simulink model "GPCA_Alarm"  (Simulink 8.7)
settings: Solver=VariableStepAuto  StartTime=0.0  StopTime=10.0  RelTol=1e-3
libraries: simulink x14
(part 1 of 3)
settings Model: Creator=bourbouh  LastModifiedBy=bourbouh
settings DataIOCC: LimitDataPoints=off  SaveFormat=Dataset
settings DebuggingCC: UnderspecifiedInitializationDetection=Simplified  MergeDetectMultiDrivingBlocksExec=error
settings HardwareCC: ProdBitPerPointer=64  ProdLargestAtomicFloat=Float  ProdIntDivRoundTo=Zero  ProdEndianess=LittleEndian  ProdWordSize=64  ProdHWDeviceType=Intel->x86-64 (Windows64)
settings ModelReferenceCC: PropagateSignalLabelsOutOfModel=on
settings ConfigComp: CovModelRefEnable=off

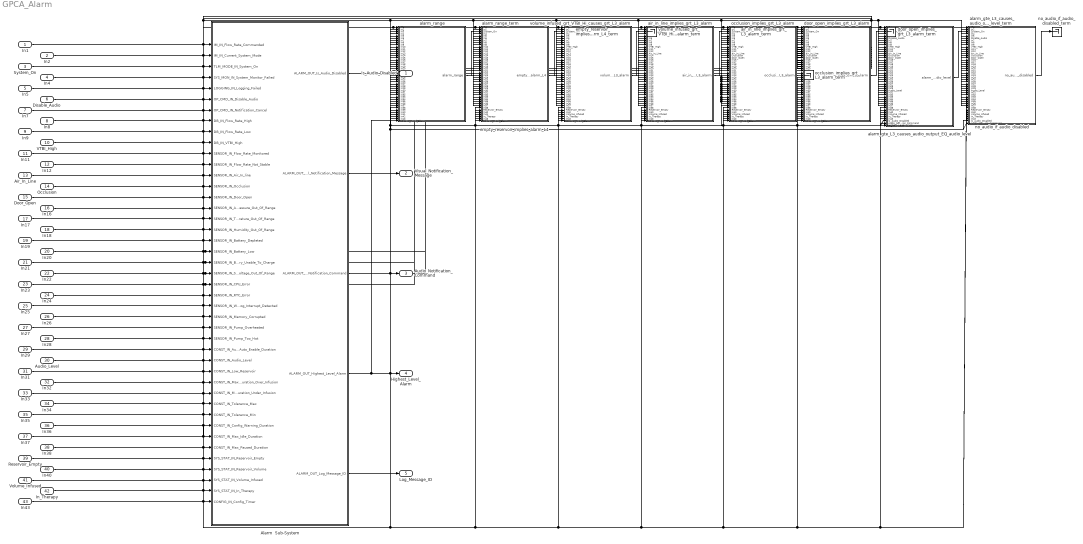
== system GPCA_Alarm ==
  In1 : Inport
  In2 : Inport  Port=2
  System_On : Inport  Port=3
  In4 : Inport  Port=4
  In5 : Inport  Port=5
  Disable_Audio : Inport  Port=6
  In7 : Inport  Port=7
  In8 : Inport  Port=8
  In9 : Inport  Port=9
  VTBI_High : Inport  Port=10
  In11 : Inport  Port=11
  In12 : Inport  Port=12
  Air_In_Line : Inport  Port=13
  Occlusion : Inport  Port=14
  Door_Open : Inport  Port=15
  In16 : Inport  Port=16
  In17 : Inport  Port=17
  In18 : Inport  Port=18
  In19 : Inport  Port=19
  In20 : Inport  Port=20
  In21 : Inport  Port=21
  In22 : Inport  Port=22
  In23 : Inport  Port=23
  In24 : Inport  Port=24
  In25 : Inport  Port=25
  In26 : Inport  Port=26
  In27 : Inport  Port=27
  In28 : Inport  Port=28
  In29 : Inport  Port=29
  Audio_Level : Inport  Port=30
  In31 : Inport  Port=31
  In32 : Inport  Port=32
  In33 : Inport  Port=33
  In34 : Inport  Port=34
  In35 : Inport  Port=35
  In36 : Inport  Port=36
  In37 : Inport  Port=37
  In38 : Inport  Port=38
  Reservoir_Empty : Inport  Port=39
  In40 : Inport  Port=40
  Volume_Infused : Inport  Port=41
  In_Therapy : Inport  Port=42
  In43 : Inport  Port=43
  Alarm  Sub-System : Stateflow chart  TreatAsAtomicUnit=on
  air_in_line_implies_grt_L3_alarm : Subsystem  TreatAsAtomicUnit=on  mask(Observer){AnnotationType=ensures, ObserverType=[]}
      mask prompts: AnnotationType "Type of annotation (pre/post...)"; ObserverType "Observer type"
      mask help:
      | Set an observer for the system.
      | The annotation type parameter sets the type of observer:
      | - requires : pre-condition
      | - ensures : post-condition
      | - assert : an assertion
      | - observer : the observer computes a special type of properties
      mask TypeOptions AnnotationType: ensures | requires | assert | observer
      mask Callback AnnotationType:
      | paramStr = get_param(gcb, 'MaskValues');
      | if strcmp(paramStr{1}(1),'o')
      | set_param(gcb,'MaskVisibilities',{'on';'on'});
      | paramStr{2} = 'ellipsoid';
      | set_param(gcb,'MaskValues',paramStr);
      | else
      | set_param(gcb,'MaskVisibilities',{'on';'off'});
      | end
      | clear paramStr;
      mask Callback ObserverType:
      | paramStr = get_param(gcb, 'MaskValues');
      | if strcmp(paramStr{1}(1),'o')
      | set_param(gcb,'MaskVisibilities',{'on';'on'});
      | paramStr{2} = 'ellipsoid';
      | set_param(gcb,'MaskValues',paramStr);
      | else
      | set_param(gcb,'MaskVisibilities',{'on';'off'});
      | end
      | clear paramStr;
      mask Display:
      | color('black')
      | text(0.5, 0.5, ['Property: ''' get_param(gcb,'name') ''''], 'horizontalAlignment', 'center');
      | text(0.99, 0.03, '{\bf\fontsize{12}TIMEOUT}', 'hor', 'right', 'ver', 'bottom', 'texmode', 'on');
  air_in_line_implies_grt_L3_alarm_term : Terminator
  alarm_gte_L3_causes_audio_output_EQ_audio_level : Subsystem  TreatAsAtomicUnit=on  mask(Observer){AnnotationType=ensures, ObserverType=[]}
      mask prompts: AnnotationType "Type of annotation (pre/post...)"; ObserverType "Observer type"
      mask help:
      | Set an observer for the system.
      | The annotation type parameter sets the type of observer:
      | - requires : pre-condition
      | - ensures : post-condition
      | - assert : an assertion
      | - observer : the observer computes a special type of properties
      mask TypeOptions AnnotationType: ensures | requires | assert | observer
      mask Callback AnnotationType:
      | paramStr = get_param(gcb, 'MaskValues');
      | if strcmp(paramStr{1}(1),'o')
      | set_param(gcb,'MaskVisibilities',{'on';'on'});
      | paramStr{2} = 'ellipsoid';
      | set_param(gcb,'MaskValues',paramStr);
      | else
      | set_param(gcb,'MaskVisibilities',{'on';'off'});
      | end
      | clear paramStr;
      mask Callback ObserverType:
      | paramStr = get_param(gcb, 'MaskValues');
      | if strcmp(paramStr{1}(1),'o')
      | set_param(gcb,'MaskVisibilities',{'on';'on'});
      | paramStr{2} = 'ellipsoid';
      | set_param(gcb,'MaskValues',paramStr);
      | else
      | set_param(gcb,'MaskVisibilities',{'on';'off'});
      | end
      | clear paramStr;
      mask Display:
      | color('red')
      | text(0.5, 0.5, ['CoCoSpec: ''' get_param(gcb,'name') ''''], 'horizontalAlignment', 'center');
      | text(0.99, 0.03, '{\bf\fontsize{12}TO BE VERIFIED}', 'hor', 'right', 'ver', 'bottom', 'texmode', 'on');
  alarm_gte_L3_causes_audio_output_EQ_audio_level_term : Terminator
  alarm_range : Subsystem  TreatAsAtomicUnit=on  mask(Observer){AnnotationType=ensures, ObserverType=[]}
      mask prompts: AnnotationType "Type of annotation (pre/post...)"; ObserverType "Observer type"
      mask help:
      | Set an observer for the system.
      | The annotation type parameter sets the type of observer:
      | - requires : pre-condition
      | - ensures : post-condition
      | - assert : an assertion
      | - observer : the observer computes a special type of properties
      mask TypeOptions AnnotationType: ensures | requires | assert | observer
      mask Callback AnnotationType:
      | paramStr = get_param(gcb, 'MaskValues');
      | if strcmp(paramStr{1}(1),'o')
      | set_param(gcb,'MaskVisibilities',{'on';'on'});
      | paramStr{2} = 'ellipsoid';
      | set_param(gcb,'MaskValues',paramStr);
      | else
      | set_param(gcb,'MaskVisibilities',{'on';'off'});
      | end
      | clear paramStr;
      mask Callback ObserverType:
      | paramStr = get_param(gcb, 'MaskValues');
      | if strcmp(paramStr{1}(1),'o')
      | set_param(gcb,'MaskVisibilities',{'on';'on'});
      | paramStr{2} = 'ellipsoid';
      | set_param(gcb,'MaskValues',paramStr);
      | else
      | set_param(gcb,'MaskVisibilities',{'on';'off'});
      | end
      | clear paramStr;
      mask Display:
      | color('black')
      | text(0.5, 0.5, ['Property: ''' get_param(gcb,'name') ''''], 'horizontalAlignment', 'center');
      | text(0.99, 0.03, '{\bf\fontsize{12}SAFE}', 'hor', 'right', 'ver', 'bottom', 'texmode', 'on');
  alarm_range_term : Terminator
  door_open_implies_grt_L3_alarm : Subsystem  TreatAsAtomicUnit=on  mask(Observer){AnnotationType=ensures, ObserverType=[]}
      mask prompts: AnnotationType "Type of annotation (pre/post...)"; ObserverType "Observer type"
      mask help:
      | Set an observer for the system.
      | The annotation type parameter sets the type of observer:
      | - requires : pre-condition
      | - ensures : post-condition
      | - assert : an assertion
      | - observer : the observer computes a special type of properties
      mask TypeOptions AnnotationType: ensures | requires | assert | observer
      mask Callback AnnotationType:
      | paramStr = get_param(gcb, 'MaskValues');
      | if strcmp(paramStr{1}(1),'o')
      | set_param(gcb,'MaskVisibilities',{'on';'on'});
      | paramStr{2} = 'ellipsoid';
      | set_param(gcb,'MaskValues',paramStr);
      | else
      | set_param(gcb,'MaskVisibilities',{'on';'off'});
      | end
      | clear paramStr;
      mask Callback ObserverType:
      | paramStr = get_param(gcb, 'MaskValues');
      | if strcmp(paramStr{1}(1),'o')
      | set_param(gcb,'MaskVisibilities',{'on';'on'});
      | paramStr{2} = 'ellipsoid';
      | set_param(gcb,'MaskValues',paramStr);
      | else
      | set_param(gcb,'MaskVisibilities',{'on';'off'});
      | end
      | clear paramStr;
      mask Display:
      | color('black')
      | text(0.5, 0.5, ['Property: ''' get_param(gcb,'name') ''''], 'horizontalAlignment', 'center');
      | text(0.99, 0.03, '{\bf\fontsize{12}TIMEOUT}', 'hor', 'right', 'ver', 'bottom', 'texmode', 'on');
  door_open_implies_grt_L3_alarm_term : Terminator
  empty_reservoir_implies_alarm_L4 : Subsystem  TreatAsAtomicUnit=on  mask(Observer){AnnotationType=ensures, ObserverType=[]}
      mask prompts: AnnotationType "Type of annotation (pre/post...)"; ObserverType "Observer type"
      mask help:
      | Set an observer for the system.
      | The annotation type parameter sets the type of observer:
      | - requires : pre-condition
      | - ensures : post-condition
      | - assert : an assertion
      | - observer : the observer computes a special type of properties
      mask TypeOptions AnnotationType: ensures | requires | assert | observer
      mask Callback AnnotationType:
      | paramStr = get_param(gcb, 'MaskValues');
      | if strcmp(paramStr{1}(1),'o')
      | set_param(gcb,'MaskVisibilities',{'on';'on'});
      | paramStr{2} = 'ellipsoid';
      | set_param(gcb,'MaskValues',paramStr);
      | else
      | set_param(gcb,'MaskVisibilities',{'on';'off'});
      | end
      | clear paramStr;
      mask Callback ObserverType:
      | paramStr = get_param(gcb, 'MaskValues');
      | if strcmp(paramStr{1}(1),'o')
      | set_param(gcb,'MaskVisibilities',{'on';'on'});
      | paramStr{2} = 'ellipsoid';
      | set_param(gcb,'MaskValues',paramStr);
      | else
      | set_param(gcb,'MaskVisibilities',{'on';'off'});
      | end
      | clear paramStr;
      mask Display:
      | color('black')
      | text(0.5, 0.5, ['Property: ''' get_param(gcb,'name') ''''], 'horizontalAlignment', 'center');
      | text(0.99, 0.03, '{\bf\fontsize{12}SAFE}', 'hor', 'right', 'ver', 'bottom', 'texmode', 'on');
  empty_reservoir_implies_alarm_L4_term : Terminator
  no_audio_if_audio_disabled : Subsystem  TreatAsAtomicUnit=on  mask(Observer){AnnotationType=ensures, ObserverType=[]}
      mask prompts: AnnotationType "Type of annotation (pre/post...)"; ObserverType "Observer type"
      mask help:
      | Set an observer for the system.
      | The annotation type parameter sets the type of observer:
      | - requires : pre-condition
      | - ensures : post-condition
      | - assert : an assertion
      | - observer : the observer computes a special type of properties
      mask TypeOptions AnnotationType: ensures | requires | assert | observer
      mask Callback AnnotationType:
      | paramStr = get_param(gcb, 'MaskValues');
      | if strcmp(paramStr{1}(1),'o')
      | set_param(gcb,'MaskVisibilities',{'on';'on'});
      | paramStr{2} = 'ellipsoid';
      | set_param(gcb,'MaskValues',paramStr);
      | else
      | set_param(gcb,'MaskVisibilities',{'on';'off'});
      | end
      | clear paramStr;
      mask Callback ObserverType:
      | paramStr = get_param(gcb, 'MaskValues');
      | if strcmp(paramStr{1}(1),'o')
      | set_param(gcb,'MaskVisibilities',{'on';'on'});
      | paramStr{2} = 'ellipsoid';
      | set_param(gcb,'MaskValues',paramStr);
      | else
      | set_param(gcb,'MaskVisibilities',{'on';'off'});
      | end
      | clear paramStr;
      mask Display:
      | color('red')
      | text(0.5, 0.5, ['CoCoSpec: ''' get_param(gcb,'name') ''''], 'horizontalAlignment', 'center');
      | text(0.99, 0.03, '{\bf\fontsize{12}TO BE VERIFIED}', 'hor', 'right', 'ver', 'bottom', 'texmode', 'on');
  no_audio_if_audio_disabled_term : Terminator
  occlusion_implies_grt_L3_alarm : Subsystem  TreatAsAtomicUnit=on  mask(Observer){AnnotationType=ensures, ObserverType=[]}
      mask prompts: AnnotationType "Type of annotation (pre/post...)"; ObserverType "Observer type"
      mask help:
      | Set an observer for the system.
      | The annotation type parameter sets the type of observer:
      | - requires : pre-condition
      | - ensures : post-condition
      | - assert : an assertion
      | - observer : the observer computes a special type of properties
      mask TypeOptions AnnotationType: ensures | requires | assert | observer
      mask Callback AnnotationType:
      | paramStr = get_param(gcb, 'MaskValues');
      | if strcmp(paramStr{1}(1),'o')
      | set_param(gcb,'MaskVisibilities',{'on';'on'});
      | paramStr{2} = 'ellipsoid';
      | set_param(gcb,'MaskValues',paramStr);
      | else
      | set_param(gcb,'MaskVisibilities',{'on';'off'});
      | end
      | clear paramStr;
      mask Callback ObserverType:
      | paramStr = get_param(gcb, 'MaskValues');
      | if strcmp(paramStr{1}(1),'o')
      | set_param(gcb,'MaskVisibilities',{'on';'on'});
      | paramStr{2} = 'ellipsoid';
      | set_param(gcb,'MaskValues',paramStr);
      | else
      | set_param(gcb,'MaskVisibilities',{'on';'off'});
      | end
      | clear paramStr;
      mask Display:
      | color('black')
      | text(0.5, 0.5, ['Property: ''' get_param(gcb,'name') ''''], 'horizontalAlignment', 'center');
      | text(0.99, 0.03, '{\bf\fontsize{12}TIMEOUT}', 'hor', 'right', 'ver', 'bottom', 'texmode', 'on');
  occlusion_implies_grt_L3_alarm_term : Terminator
  volume_infused_grt_VTBI_Hi_causes_grt_L3_alarm : Subsystem  TreatAsAtomicUnit=on  mask(Observer){AnnotationType=ensures, ObserverType=[]}
      mask prompts: AnnotationType "Type of annotation (pre/post...)"; ObserverType "Observer type"
      mask help:
      | Set an observer for the system.
      | The annotation type parameter sets the type of observer:
      | - requires : pre-condition
      | - ensures : post-condition
      | - assert : an assertion
      | - observer : the observer computes a special type of properties
      mask TypeOptions AnnotationType: ensures | requires | assert | observer
      mask Callback AnnotationType:
      | paramStr = get_param(gcb, 'MaskValues');
      | if strcmp(paramStr{1}(1),'o')
      | set_param(gcb,'MaskVisibilities',{'on';'on'});
      | paramStr{2} = 'ellipsoid';
      | set_param(gcb,'MaskValues',paramStr);
      | else
      | set_param(gcb,'MaskVisibilities',{'on';'off'});
      | end
      | clear paramStr;
      mask Callback ObserverType:
      | paramStr = get_param(gcb, 'MaskValues');
      | if strcmp(paramStr{1}(1),'o')
      | set_param(gcb,'MaskVisibilities',{'on';'on'});
      | paramStr{2} = 'ellipsoid';
      | set_param(gcb,'MaskValues',paramStr);
      | else
      | set_param(gcb,'MaskVisibilities',{'on';'off'});
      | end
      | clear paramStr;
      mask Display:
      | color('black')
      | text(0.5, 0.5, ['Property: ''' get_param(gcb,'name') ''''], 'horizontalAlignment', 'center');
      | text(0.99, 0.03, '{\bf\fontsize{12}SAFE}', 'hor', 'right', 'ver', 'bottom', 'texmode', 'on');
  volume_infused_grt_VTBI_Hi_causes_grt_L3_alarm_term : Terminator
  Is_Audio_Disabled : Outport
  Visual_Notification_Message : Outport  Port=2
  Audio_Notification_Command : Outport  Port=3
  Highest_Level_Alarm : Outport  Port=4
  Log_Message_ID : Outport  Port=5
  wires:
  In1/1 -> alarm_gte_L3_causes_audio_output_EQ_audio_level/1(In1), no_audio_if_audio_disabled/1(In1), door_open_implies_grt_L3_alarm/1(In1), occlusion_implies_grt_L3_alarm/1(In1), air_in_line_implies_grt_L3_alarm/1(In1), volume_infused_grt_VTBI_Hi_causes_grt_L3_alarm/1(In1), empty_reservoir_implies_alarm_L4/1(In1), alarm_range/1(In1), Alarm  Sub-System/1(IM_IN_Flow_Rate_Commanded)
  In2/1 -> alarm_gte_L3_causes_audio_output_EQ_audio_level/2(In2), no_audio_if_audio_disabled/2(In2), occlusion_implies_grt_L3_alarm/2(In2), air_in_line_implies_grt_L3_alarm/2(In2), volume_infused_grt_VTBI_Hi_causes_grt_L3_alarm/2(In2), empty_reservoir_implies_alarm_L4/2(In2), alarm_range/2(In2), door_open_implies_grt_L3_alarm/2(In2), Alarm  Sub-System/2(IM_IN_Current_System_Mode)
  System_On/1 -> alarm_gte_L3_causes_audio_output_EQ_audio_level/3(System_On), no_audio_if_audio_disabled/3(System_On), occlusion_implies_grt_L3_alarm/3(System_On), air_in_line_implies_grt_L3_alarm/3(System_On), volume_infused_grt_VTBI_Hi_causes_grt_L3_alarm/3(System_On), empty_reservoir_implies_alarm_L4/3(System_On), alarm_range/3(In3), door_open_implies_grt_L3_alarm/3(System_On), Alarm  Sub-System/3(TLM_MODE_IN_System_On)
  In4/1 -> alarm_gte_L3_causes_audio_output_EQ_audio_level/4(In4), no_audio_if_audio_disabled/4(In4), occlusion_implies_grt_L3_alarm/4(In4), air_in_line_implies_grt_L3_alarm/4(In4), volume_infused_grt_VTBI_Hi_causes_grt_L3_alarm/4(In4), empty_reservoir_implies_alarm_L4/4(In4), alarm_range/4(In4), door_open_implies_grt_L3_alarm/4(In4), Alarm  Sub-System/4(SYS_MON_IN_System_Monitor_Failed)
  In5/1 -> alarm_gte_L3_causes_audio_output_EQ_audio_level/5(In5), no_audio_if_audio_disabled/5(In5), occlusion_implies_grt_L3_alarm/5(In5), air_in_line_implies_grt_L3_alarm/5(In5), volume_infused_grt_VTBI_Hi_causes_grt_L3_alarm/5(In5), empty_reservoir_implies_alarm_L4/5(In5), alarm_range/5(In5), door_open_implies_grt_L3_alarm/5(In5), Alarm  Sub-System/5(LOGGING_IN_Logging_Failed)
  Disable_Audio/1 -> alarm_gte_L3_causes_audio_output_EQ_audio_level/6(Disable_Audio), no_audio_if_audio_disabled/6(Disable_Audio), occlusion_implies_grt_L3_alarm/6(In6), air_in_line_implies_grt_L3_alarm/6(In6), volume_infused_grt_VTBI_Hi_causes_grt_L3_alarm/6(In6), empty_reservoir_implies_alarm_L4/6(In6), alarm_range/6(In6), door_open_implies_grt_L3_alarm/6(In6), Alarm  Sub-System/6(OP_CMD_IN_Disable_Audio)
  In7/1 -> alarm_gte_L3_causes_audio_output_EQ_audio_level/7(In7), no_audio_if_audio_disabled/7(In7), occlusion_implies_grt_L3_alarm/7(In7), air_in_line_implies_grt_L3_alarm/7(In7), volume_infused_grt_VTBI_Hi_causes_grt_L3_alarm/7(In7), empty_reservoir_implies_alarm_L4/7(In7), alarm_range/7(In7), door_open_implies_grt_L3_alarm/7(In7), Alarm  Sub-System/7(OP_CMD_IN_Notification_Cancel)
  In8/1 -> alarm_gte_L3_causes_audio_output_EQ_audio_level/8(In8), no_audio_if_audio_disabled/8(In8), occlusion_implies_grt_L3_alarm/8(In8), air_in_line_implies_grt_L3_alarm/8(In8), volume_infused_grt_VTBI_Hi_causes_grt_L3_alarm/8(In8), empty_reservoir_implies_alarm_L4/8(In8), alarm_range/8(In8), door_open_implies_grt_L3_alarm/8(In8), Alarm  Sub-System/8(DB_IN_Flow_Rate_High)
  In9/1 -> alarm_gte_L3_causes_audio_output_EQ_audio_level/9(In9), no_audio_if_audio_disabled/9(In9), door_open_implies_grt_L3_alarm/9(In9), occlusion_implies_grt_L3_alarm/9(In9), air_in_line_implies_grt_L3_alarm/9(In9), volume_infused_grt_VTBI_Hi_causes_grt_L3_alarm/9(In9), empty_reservoir_implies_alarm_L4/9(In9), alarm_range/9(In9), Alarm  Sub-System/9(DB_IN_Flow_Rate_Low)
  VTBI_High/1 -> alarm_gte_L3_causes_audio_output_EQ_audio_level/10(VTBI_High), no_audio_if_audio_disabled/10(VTBI_High), door_open_implies_grt_L3_alarm/10(VTBI_High), occlusion_implies_grt_L3_alarm/10(VTBI_High), air_in_line_implies_grt_L3_alarm/10(VTBI_High), volume_infused_grt_VTBI_Hi_causes_grt_L3_alarm/10(VTBI_High), empty_reservoir_implies_alarm_L4/10(In10), alarm_range/10(In10), Alarm  Sub-System/10(DB_IN_VTBI_High)
  In11/1 -> alarm_gte_L3_causes_audio_output_EQ_audio_level/11(In11), no_audio_if_audio_disabled/11(In11), door_open_implies_grt_L3_alarm/11(In11), occlusion_implies_grt_L3_alarm/11(In11), air_in_line_implies_grt_L3_alarm/11(In11), volume_infused_grt_VTBI_Hi_causes_grt_L3_alarm/11(In11), empty_reservoir_implies_alarm_L4/11(In11), alarm_range/11(In11), Alarm  Sub-System/11(SENSOR_IN_Flow_Rate_Monitored)
  In12/1 -> alarm_gte_L3_causes_audio_output_EQ_audio_level/12(In12), no_audio_if_audio_disabled/12(In12), door_open_implies_grt_L3_alarm/12(In12), occlusion_implies_grt_L3_alarm/12(In12), air_in_line_implies_grt_L3_alarm/12(In12), volume_infused_grt_VTBI_Hi_causes_grt_L3_alarm/12(In12), empty_reservoir_implies_alarm_L4/12(In12), alarm_range/12(In12), Alarm  Sub-System/12(SENSOR_IN_Flow_Rate_Not_Stable)
  Air_In_Line/1 -> alarm_gte_L3_causes_audio_output_EQ_audio_level/13(Air_In_Line), no_audio_if_audio_disabled/13(Air_In_Line), door_open_implies_grt_L3_alarm/13(Air_In_Line), occlusion_implies_grt_L3_alarm/13(Air_In_Line), air_in_line_implies_grt_L3_alarm/13(Air_In_Line), volume_infused_grt_VTBI_Hi_causes_grt_L3_alarm/13(In13), empty_reservoir_implies_alarm_L4/13(In13), alarm_range/13(In13), Alarm  Sub-System/13(SENSOR_IN_Air_In_line)
  Occlusion/1 -> alarm_gte_L3_causes_audio_output_EQ_audio_level/14(Occlusion), no_audio_if_audio_disabled/14(Occlusion), door_open_implies_grt_L3_alarm/14(Occlusion), occlusion_implies_grt_L3_alarm/14(Occlusion), air_in_line_implies_grt_L3_alarm/14(In14), volume_infused_grt_VTBI_Hi_causes_grt_L3_alarm/14(In14), empty_reservoir_implies_alarm_L4/14(In14), alarm_range/14(In14), Alarm  Sub-System/14(SENSOR_IN_Occlusion)
  Door_Open/1 -> alarm_gte_L3_causes_audio_output_EQ_audio_level/15(Door_Open), no_audio_if_audio_disabled/15(Door_Open), door_open_implies_grt_L3_alarm/15(Door_Open), occlusion_implies_grt_L3_alarm/15(Door_Open), air_in_line_implies_grt_L3_alarm/15(In15), volume_infused_grt_VTBI_Hi_causes_grt_L3_alarm/15(In15), empty_reservoir_implies_alarm_L4/15(In15), alarm_range/15(In15), Alarm  Sub-System/15(SENSOR_IN_Door_Open)
  In16/1 -> alarm_gte_L3_causes_audio_output_EQ_audio_level/16(In16), no_audio_if_audio_disabled/16(In16), door_open_implies_grt_L3_alarm/16(In16), occlusion_implies_grt_L3_alarm/16(In16), air_in_line_implies_grt_L3_alarm/16(In16), volume_infused_grt_VTBI_Hi_causes_grt_L3_alarm/16(In16), empty_reservoir_implies_alarm_L4/16(In16), alarm_range/16(In16), Alarm  Sub-System/16(SENSOR_IN_Air_Pressure_Out_Of_Range)
  In17/1 -> alarm_gte_L3_causes_audio_output_EQ_audio_level/17(In17), no_audio_if_audio_disabled/17(In17), door_open_implies_grt_L3_alarm/17(In17), occlusion_implies_grt_L3_alarm/17(In17), air_in_line_implies_grt_L3_alarm/17(In17), volume_infused_grt_VTBI_Hi_causes_grt_L3_alarm/17(In17), empty_reservoir_implies_alarm_L4/17(In17), alarm_range/17(In17), Alarm  Sub-System/17(SENSOR_IN_Temperature_Out_Of_Range)
  In18/1 -> alarm_gte_L3_causes_audio_output_EQ_audio_level/18(In18), no_audio_if_audio_disabled/18(In18), door_open_implies_grt_L3_alarm/18(In18), occlusion_implies_grt_L3_alarm/18(In18), air_in_line_implies_grt_L3_alarm/18(In18), volume_infused_grt_VTBI_Hi_causes_grt_L3_alarm/18(In18), empty_reservoir_implies_alarm_L4/18(In18), alarm_range/18(In18), Alarm  Sub-System/18(SENSOR_IN_Humidity_Out_Of_Range)
  In19/1 -> alarm_gte_L3_causes_audio_output_EQ_audio_level/19(In19), no_audio_if_audio_disabled/19(In19), door_open_implies_grt_L3_alarm/19(In19), occlusion_implies_grt_L3_alarm/19(In19), air_in_line_implies_grt_L3_alarm/19(In19), volume_infused_grt_VTBI_Hi_causes_grt_L3_alarm/19(In19), empty_reservoir_implies_alarm_L4/19(In19), alarm_range/19(In19), Alarm  Sub-System/19(SENSOR_IN_Battery_Depleted)
  In20/1 -> door_open_implies_grt_L3_alarm/20(In20), Alarm  Sub-System/20(SENSOR_IN_Battery_Low), alarm_gte_L3_causes_audio_output_EQ_audio_level/20(In20), no_audio_if_audio_disabled/20(In20), occlusion_implies_grt_L3_alarm/20(In20), air_in_line_implies_grt_L3_alarm/20(In20), volume_infused_grt_VTBI_Hi_causes_grt_L3_alarm/20(In20), empty_reservoir_implies_alarm_L4/20(In20), alarm_range/20(In20)
  In21/1 -> door_open_implies_grt_L3_alarm/21(In21), Alarm  Sub-System/21(SENSOR_IN_Battery_Unable_To_Charge), alarm_gte_L3_causes_audio_output_EQ_audio_level/21(In21), no_audio_if_audio_disabled/21(In21), occlusion_implies_grt_L3_alarm/21(In21), air_in_line_implies_grt_L3_alarm/21(In21), volume_infused_grt_VTBI_Hi_causes_grt_L3_alarm/21(In21), empty_reservoir_implies_alarm_L4/21(In21), alarm_range/21(In21)
  In22/1 -> door_open_implies_grt_L3_alarm/22(In22), Alarm  Sub-System/22(SENSOR_IN_Supply_Voltage_Out_Of_Range), alarm_gte_L3_causes_audio_output_EQ_audio_level/22(In22), no_audio_if_audio_disabled/22(In22), occlusion_implies_grt_L3_alarm/22(In22), air_in_line_implies_grt_L3_alarm/22(In22), volume_infused_grt_VTBI_Hi_causes_grt_L3_alarm/22(In22), empty_reservoir_implies_alarm_L4/22(In22), alarm_range/22(In22)
  In23/1 -> door_open_implies_grt_L3_alarm/23(In23), Alarm  Sub-System/23(SENSOR_IN_CPU_Error), alarm_gte_L3_causes_audio_output_EQ_audio_level/23(In23), no_audio_if_audio_disabled/23(In23), occlusion_implies_grt_L3_alarm/23(In23), air_in_line_implies_grt_L3_alarm/23(In23), volume_infused_grt_VTBI_Hi_causes_grt_L3_alarm/23(In23), empty_reservoir_implies_alarm_L4/23(In23), alarm_range/23(In23)
  In24/1 -> occlusion_implies_grt_L3_alarm/24(In24), door_open_implies_grt_L3_alarm/24(In24), alarm_gte_L3_causes_audio_output_EQ_audio_level/24(In24), no_audio_if_audio_disabled/24(In24), air_in_line_implies_grt_L3_alarm/24(In24), volume_infused_grt_VTBI_Hi_causes_grt_L3_alarm/24(In24), empty_reservoir_implies_alarm_L4/24(In24), alarm_range/24(In24), Alarm  Sub-System/24(SENSOR_IN_RTC_Error)
  In25/1 -> occlusion_implies_grt_L3_alarm/25(In25), door_open_implies_grt_L3_alarm/25(In25), alarm_gte_L3_causes_audio_output_EQ_audio_level/25(In25), no_audio_if_audio_disabled/25(In25), air_in_line_implies_grt_L3_alarm/25(In25), volume_infused_grt_VTBI_Hi_causes_grt_L3_alarm/25(In25), empty_reservoir_implies_alarm_L4/25(In25), alarm_range/25(In25), Alarm  Sub-System/25(SENSOR_IN_WatchDog_Interrupt_Detected)
  In26/1 -> occlusion_implies_grt_L3_alarm/26(In26), door_open_implies_grt_L3_alarm/26(In26), alarm_gte_L3_causes_audio_output_EQ_audio_level/26(In26), no_audio_if_audio_disabled/26(In26), air_in_line_implies_grt_L3_alarm/26(In26), volume_infused_grt_VTBI_Hi_causes_grt_L3_alarm/26(In26), empty_reservoir_implies_alarm_L4/26(In26), alarm_range/26(In26), Alarm  Sub-System/26(SENSOR_IN_Memory_Corrupted)
  In27/1 -> occlusion_implies_grt_L3_alarm/27(In27), door_open_implies_grt_L3_alarm/27(In27), alarm_gte_L3_causes_audio_output_EQ_audio_level/27(In27), no_audio_if_audio_disabled/27(In27), air_in_line_implies_grt_L3_alarm/27(In27), volume_infused_grt_VTBI_Hi_causes_grt_L3_alarm/27(In27), empty_reservoir_implies_alarm_L4/27(In27), alarm_range/27(In27), Alarm  Sub-System/27(SENSOR_IN_Pump_Overheated)
  In28/1 -> occlusion_implies_grt_L3_alarm/28(In28), door_open_implies_grt_L3_alarm/28(In28), alarm_gte_L3_causes_audio_output_EQ_audio_level/28(In28), no_audio_if_audio_disabled/28(In28), air_in_line_implies_grt_L3_alarm/28(In28), volume_infused_grt_VTBI_Hi_causes_grt_L3_alarm/28(In28), empty_reservoir_implies_alarm_L4/28(In28), alarm_range/28(In28), Alarm  Sub-System/28(SENSOR_IN_Pump_Too_Hot)
  In29/1 -> occlusion_implies_grt_L3_alarm/29(In29), door_open_implies_grt_L3_alarm/29(In29), alarm_gte_L3_causes_audio_output_EQ_audio_level/29(In29), no_audio_if_audio_disabled/29(In29), air_in_line_implies_grt_L3_alarm/29(In29), volume_infused_grt_VTBI_Hi_causes_grt_L3_alarm/29(In29), empty_reservoir_implies_alarm_L4/29(In29), alarm_range/29(In29), Alarm  Sub-System/29(CONST_IN_Audio_Auto_Enable_Duration)
  Audio_Level/1 -> occlusion_implies_grt_L3_alarm/30(In30), door_open_implies_grt_L3_alarm/30(In30), alarm_gte_L3_causes_audio_output_EQ_audio_level/30(Audio_Level), no_audio_if_audio_disabled/30(Audio_Level), air_in_line_implies_grt_L3_alarm/30(In30), volume_infused_grt_VTBI_Hi_causes_grt_L3_alarm/30(In30), empty_reservoir_implies_alarm_L4/30(In30), alarm_range/30(In30), Alarm  Sub-System/30(CONST_IN_Audio_Level)
  In31/1 -> occlusion_implies_grt_L3_alarm/31(In31), door_open_implies_grt_L3_alarm/31(In31), alarm_gte_L3_causes_audio_output_EQ_audio_level/31(In31), no_audio_if_audio_disabled/31(In31), air_in_line_implies_grt_L3_alarm/31(In31), volume_infused_grt_VTBI_Hi_causes_grt_L3_alarm/31(In31), empty_reservoir_implies_alarm_L4/31(In31), alarm_range/31(In31), Alarm  Sub-System/31(CONST_IN_Low_Reservoir)
  In32/1 -> occlusion_implies_grt_L3_alarm/32(In32), door_open_implies_grt_L3_alarm/32(In32), alarm_gte_L3_causes_audio_output_EQ_audio_level/32(In32), no_audio_if_audio_disabled/32(In32), air_in_line_implies_grt_L3_alarm/32(In32), volume_infused_grt_VTBI_Hi_causes_grt_L3_alarm/32(In32), empty_reservoir_implies_alarm_L4/32(In32), alarm_range/32(In32), Alarm  Sub-System/32(CONST_IN_Max_Duration_Over_Infusion)
  In33/1 -> occlusion_implies_grt_L3_alarm/33(In33), door_open_implies_grt_L3_alarm/33(In33), alarm_gte_L3_causes_audio_output_EQ_audio_level/33(In33), no_audio_if_audio_disabled/33(In33), air_in_line_implies_grt_L3_alarm/33(In33), volume_infused_grt_VTBI_Hi_causes_grt_L3_alarm/33(In33), empty_reservoir_implies_alarm_L4/33(In33), alarm_range/33(In33), Alarm  Sub-System/33(CONST_IN_Max_Duration_Under_Infusion)
  In34/1 -> occlusion_implies_grt_L3_alarm/34(In34), door_open_implies_grt_L3_alarm/34(In34), alarm_gte_L3_causes_audio_output_EQ_audio_level/34(In34), no_audio_if_audio_disabled/34(In34), air_in_line_implies_grt_L3_alarm/34(In34), volume_infused_grt_VTBI_Hi_causes_grt_L3_alarm/34(In34), empty_reservoir_implies_alarm_L4/34(In34), alarm_range/34(In34), Alarm  Sub-System/34(CONST_IN_Tolerance_Max)
  In35/1 -> occlusion_implies_grt_L3_alarm/35(In35), door_open_implies_grt_L3_alarm/35(In35), alarm_gte_L3_causes_audio_output_EQ_audio_level/35(In35), no_audio_if_audio_disabled/35(In35), air_in_line_implies_grt_L3_alarm/35(In35), volume_infused_grt_VTBI_Hi_causes_grt_L3_alarm/35(In35), empty_reservoir_implies_alarm_L4/35(In35), alarm_range/35(In35), Alarm  Sub-System/35(CONST_IN_Tolerance_Min)
  In36/1 -> alarm_gte_L3_causes_audio_output_EQ_audio_level/36(In36), no_audio_if_audio_disabled/36(In36), occlusion_implies_grt_L3_alarm/36(In36), air_in_line_implies_grt_L3_alarm/36(In36), volume_infused_grt_VTBI_Hi_causes_grt_L3_alarm/36(In36), empty_reservoir_implies_alarm_L4/36(In36), alarm_range/36(In36), door_open_implies_grt_L3_alarm/36(In36), Alarm  Sub-System/36(CONST_IN_Config_Warning_Duration)
  In37/1 -> alarm_gte_L3_causes_audio_output_EQ_audio_level/37(In37), no_audio_if_audio_disabled/37(In37), occlusion_implies_grt_L3_alarm/37(In37), air_in_line_implies_grt_L3_alarm/37(In37), volume_infused_grt_VTBI_Hi_causes_grt_L3_alarm/37(In37), empty_reservoir_implies_alarm_L4/37(In37), alarm_range/37(In37), door_open_implies_grt_L3_alarm/37(In37), Alarm  Sub-System/37(CONST_IN_Max_Idle_Duration)
  In38/1 -> alarm_gte_L3_causes_audio_output_EQ_audio_level/38(In38), no_audio_if_audio_disabled/38(In38), door_open_implies_grt_L3_alarm/38(In38), occlusion_implies_grt_L3_alarm/38(In38), air_in_line_implies_grt_L3_alarm/38(In38), volume_infused_grt_VTBI_Hi_causes_grt_L3_alarm/38(In38), empty_reservoir_implies_alarm_L4/38(In38), alarm_range/38(In38), Alarm  Sub-System/38(CONST_IN_Max_Paused_Duration)
  Reservoir_Empty/1 -> alarm_gte_L3_causes_audio_output_EQ_audio_level/39(Reservoir_Empty), no_audio_if_audio_disabled/39(Reservoir_Empty), door_open_implies_grt_L3_alarm/39(Reservoir_Empty), occlusion_implies_grt_L3_alarm/39(Reservoir_Empty), air_in_line_implies_grt_L3_alarm/39(Reservoir_Empty), volume_infused_grt_VTBI_Hi_causes_grt_L3_alarm/39(Reservoir_Empty), empty_reservoir_implies_alarm_L4/39(Reservoir_Empty), alarm_range/39(In39), Alarm  Sub-System/39(SYS_STAT_IN_Reservoir_Empty)
  In40/1 -> alarm_gte_L3_causes_audio_output_EQ_audio_level/40(In40), no_audio_if_audio_disabled/40(In40), door_open_implies_grt_L3_alarm/40(In40), occlusion_implies_grt_L3_alarm/40(In40), air_in_line_implies_grt_L3_alarm/40(In40), volume_infused_grt_VTBI_Hi_causes_grt_L3_alarm/40(In40), empty_reservoir_implies_alarm_L4/40(In40), alarm_range/40(In40), Alarm  Sub-System/40(SYS_STAT_IN_Reservoir_Volume)
  Volume_Infused/1 -> alarm_gte_L3_causes_audio_output_EQ_audio_level/41(Volume_Infused), no_audio_if_audio_disabled/41(Volume_Infused), door_open_implies_grt_L3_alarm/41(Volume_Infused), occlusion_implies_grt_L3_alarm/41(Volume_Infused), air_in_line_implies_grt_L3_alarm/41(Volume_Infused), volume_infused_grt_VTBI_Hi_causes_grt_L3_alarm/41(Volume_Infused), empty_reservoir_implies_alarm_L4/41(In41), alarm_range/41(In41), Alarm  Sub-System/41(SYS_STAT_IN_Volume_Infused)
  In_Therapy/1 -> alarm_gte_L3_causes_audio_output_EQ_audio_level/42(In_Therapy), no_audio_if_audio_disabled/42(In_Therapy), door_open_implies_grt_L3_alarm/42(In_Therapy), occlusion_implies_grt_L3_alarm/42(In_Therapy), air_in_line_implies_grt_L3_alarm/42(In_Therapy), volume_infused_grt_VTBI_Hi_causes_grt_L3_alarm/42(In_Therapy), empty_reservoir_implies_alarm_L4/42(In_Therapy), alarm_range/42(In42), Alarm  Sub-System/42(SYS_STAT_IN_In_Therapy)
  In43/1 -> alarm_gte_L3_causes_audio_output_EQ_audio_level/43(In43), no_audio_if_audio_disabled/43(In43), door_open_implies_grt_L3_alarm/43(In43), occlusion_implies_grt_L3_alarm/43(In43), air_in_line_implies_grt_L3_alarm/43(In43), volume_infused_grt_VTBI_Hi_causes_grt_L3_alarm/43(In43), empty_reservoir_implies_alarm_L4/43(In43), alarm_range/43(In43), Alarm  Sub-System/43(CONFIG_IN_Config_Timer)
  Alarm  Sub-System/1(ALARM_OUT_Is_Audio_Disabled) -> alarm_gte_L3_causes_audio_output_EQ_audio_level/44(Is_Audio_Disabled), no_audio_if_audio_disabled/44(Is_Audio_Disabled), Is_Audio_Disabled/1
  Alarm  Sub-System/2(ALARM_OUT_Visual_Notification_Message) -> Visual_Notification_Message/1
  Alarm  Sub-System/3(ALARM_OUT_Audio_Notification_Command) -> alarm_gte_L3_causes_audio_output_EQ_audio_level/45(Audio_Notification_Command), no_audio_if_audio_disabled/45(Audio_Notification_Command), Audio_Notification_Command/1
  Alarm  Sub-System/4(ALARM_OUT_Highest_Level_Alarm) -> door_open_implies_grt_L3_alarm/44(Highest_Level_Alarm), alarm_gte_L3_causes_audio_output_EQ_audio_level/46(Highest_Level_Alarm), occlusion_implies_grt_L3_alarm/44(Highest_Level_Alarm), air_in_line_implies_grt_L3_alarm/44(Highest_Level_Alarm), volume_infused_grt_VTBI_Hi_causes_grt_L3_alarm/44(Highest_Level_Alarm), empty_reservoir_implies_alarm_L4/44(Highest_Level_Alarm), Highest_Level_Alarm/1, alarm_range/44(Highest_Level_Alarm)
  Alarm  Sub-System/5(ALARM_OUT_Log_Message_ID) -> Log_Message_ID/1
  alarm_range/1(alarm_range) -> alarm_range_term/1
  empty_reservoir_implies_alarm_L4/1(empty_reservoir_implies_alarm_L4) -> empty_reservoir_implies_alarm_L4_term/1
  volume_infused_grt_VTBI_Hi_causes_grt_L3_alarm/1(volume_infused_grt_VTBI_Hi_causes_grt_L3_alarm) -> volume_infused_grt_VTBI_Hi_causes_grt_L3_alarm_term/1
  air_in_line_implies_grt_L3_alarm/1(air_in_line_implies_grt_L3_alarm) -> air_in_line_implies_grt_L3_alarm_term/1
  occlusion_implies_grt_L3_alarm/1(occlusion_implies_grt_L3_alarm) -> occlusion_implies_grt_L3_alarm_term/1
  door_open_implies_grt_L3_alarm/1(door_open_implies_grt_L3_alarm) -> door_open_implies_grt_L3_alarm_term/1
  alarm_gte_L3_causes_audio_output_EQ_audio_level/1(alarm_gte_L3_causes_audio_output_EQ_audio_level) -> alarm_gte_L3_causes_audio_output_EQ_audio_level_term/1
  no_audio_if_audio_disabled/1(no_audio_if_audio_disabled) -> no_audio_if_audio_disabled_term/1

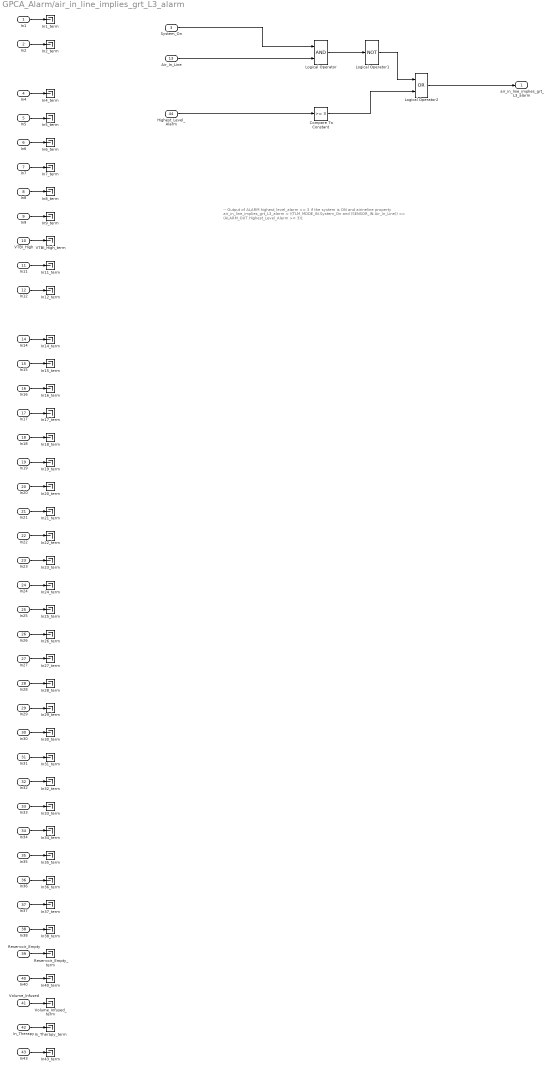
== system GPCA_Alarm/air_in_line_implies_grt_L3_alarm ==
  note: -- Output of ALARM highest_level_alarm >= 3 if the system is ON and airineline
      | property air_in_line_implies_grt_L3_alarm =
      | ((TLM_MODE_IN.System_On and (SENSOR_IN.Air_In_Line)) => (ALARM_OUT.Highest_Level_Alarm >= 3));
  In1 : Inport
  In2 : Inport  Port=2
  System_On : Inport  Port=3
  In4 : Inport  Port=4
  In5 : Inport  Port=5
  In6 : Inport  Port=6
  In7 : Inport  Port=7
  In8 : Inport  Port=8
  In9 : Inport  Port=9
  VTBI_High : Inport  Port=10
  In11 : Inport  Port=11
  In12 : Inport  Port=12
  Air_In_Line : Inport  Port=13
  In14 : Inport  Port=14
  In15 : Inport  Port=15
  In16 : Inport  Port=16
  In17 : Inport  Port=17
  In18 : Inport  Port=18
  In19 : Inport  Port=19
  In20 : Inport  Port=20
  In21 : Inport  Port=21
  In22 : Inport  Port=22
  In23 : Inport  Port=23
  In24 : Inport  Port=24
  In25 : Inport  Port=25
  In26 : Inport  Port=26
  In27 : Inport  Port=27
  In28 : Inport  Port=28
  In29 : Inport  Port=29
  In30 : Inport  Port=30
  In31 : Inport  Port=31
  In32 : Inport  Port=32
  In33 : Inport  Port=33
  In34 : Inport  Port=34
  In35 : Inport  Port=35
  In36 : Inport  Port=36
  In37 : Inport  Port=37
  In38 : Inport  Port=38
  Reservoir_Empty : Inport  Port=39
  In40 : Inport  Port=40
  Volume_Infused : Inport  Port=41
  In_Therapy : Inport  Port=42
  In43 : Inport  Port=43
  Highest_Level_Alarm : Inport  Port=44
  Compare To Constant : simulink/Logic and Bit Operations/Compare To Constant  relop=>=  const=3  OutDataTypeStr=boolean
  In11_term : Terminator
  In12_term : Terminator
  In14_term : Terminator
  In15_term : Terminator
  In16_term : Terminator
  In17_term : Terminator
  In18_term : Terminator
  In19_term : Terminator
  In1_term : Terminator
  In20_term : Terminator
  In21_term : Terminator
  In22_term : Terminator
  In23_term : Terminator
  In24_term : Terminator
  In25_term : Terminator
  In26_term : Terminator
  In27_term : Terminator
  In28_term : Terminator
  In29_term : Terminator
  In2_term : Terminator
  In30_term : Terminator
  In31_term : Terminator
  In32_term : Terminator
  In33_term : Terminator
  In34_term : Terminator
  In35_term : Terminator
  In36_term : Terminator
  In37_term : Terminator
  In38_term : Terminator
  In40_term : Terminator
  In43_term : Terminator
  In4_term : Terminator
  In5_term : Terminator
  In6_term : Terminator
  In7_term : Terminator
  In8_term : Terminator
  In9_term : Terminator
  In_Therapy_term : Terminator
  Logical Operator : Logic  AllPortsSameDT=off  OutDataTypeStr=boolean
  Logical Operator1 : Logic  Operator=NOT  Inputs=3  AllPortsSameDT=off  OutDataTypeStr=boolean
  Logical Operator2 : Logic  Operator=OR  AllPortsSameDT=off  OutDataTypeStr=boolean
  Reservoir_Empty_term : Terminator
  VTBI_High_term : Terminator
  Volume_Infused_term : Terminator
  air_in_line_implies_grt_L3_alarm : Outport
  wires:
  In1/1 -> In1_term/1
  In2/1 -> In2_term/1
  In4/1 -> In4_term/1
  In5/1 -> In5_term/1
  In6/1 -> In6_term/1
  In7/1 -> In7_term/1
  In8/1 -> In8_term/1
  In9/1 -> In9_term/1
  VTBI_High/1 -> VTBI_High_term/1
  In11/1 -> In11_term/1
  In12/1 -> In12_term/1
  In14/1 -> In14_term/1
  In15/1 -> In15_term/1
  In16/1 -> In16_term/1
  In17/1 -> In17_term/1
  In18/1 -> In18_term/1
  In19/1 -> In19_term/1
  In20/1 -> In20_term/1
  In21/1 -> In21_term/1
  In22/1 -> In22_term/1
  In23/1 -> In23_term/1
  In24/1 -> In24_term/1
  In25/1 -> In25_term/1
  In26/1 -> In26_term/1
  In27/1 -> In27_term/1
  In28/1 -> In28_term/1
  In29/1 -> In29_term/1
  In30/1 -> In30_term/1
  In31/1 -> In31_term/1
  In32/1 -> In32_term/1
  In33/1 -> In33_term/1
  In34/1 -> In34_term/1
  In35/1 -> In35_term/1
  In36/1 -> In36_term/1
  In37/1 -> In37_term/1
  In38/1 -> In38_term/1
  Reservoir_Empty/1 -> Reservoir_Empty_term/1
  In40/1 -> In40_term/1
  Volume_Infused/1 -> Volume_Infused_term/1
  In_Therapy/1 -> In_Therapy_term/1
  In43/1 -> In43_term/1
  System_On/1 -> Logical Operator/1
  Air_In_Line/1 -> Logical Operator/2
  Highest_Level_Alarm/1 -> Compare To Constant/1
  Logical Operator/1 -> Logical Operator1/1
  Logical Operator1/1 -> Logical Operator2/1
  Compare To Constant/1 -> Logical Operator2/2
  Logical Operator2/1 -> air_in_line_implies_grt_L3_alarm/1

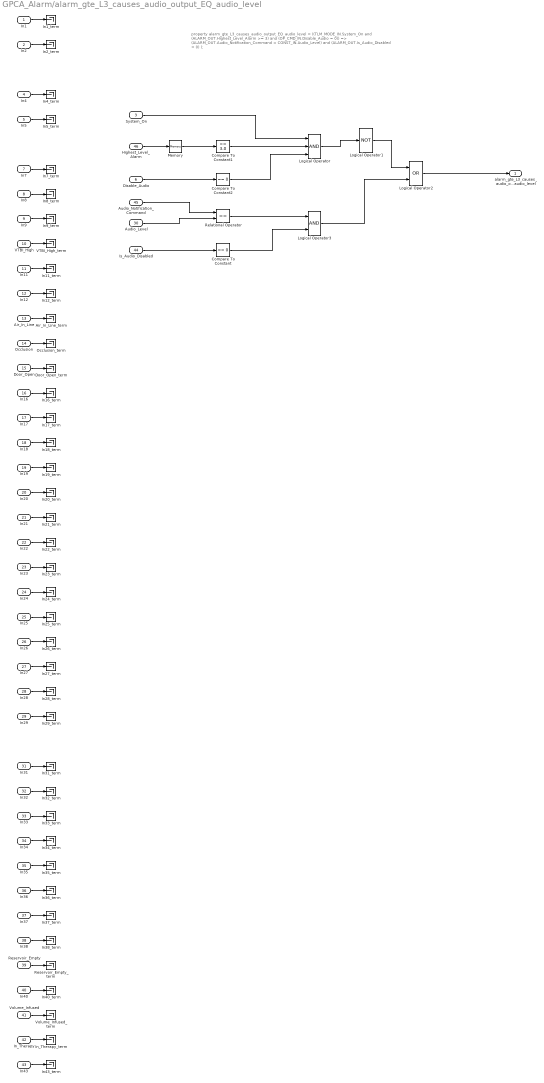
== system GPCA_Alarm/alarm_gte_L3_causes_audio_output_EQ_audio_level ==
  note: property alarm_gte_L3_causes_audio_output_EQ_audio_level =
      | ((TLM_MODE_IN.System_On and (ALARM_OUT.Highest_Level_Alarm >= 3) and (OP_CMD_IN.Disable_Audio = 0))
      | => (ALARM_OUT.Audio_Notification_Command = CONST_IN.Audio_Level) and (ALARM_OUT.Is_Audio_Disabled = 0) );
  In1 : Inport
  In2 : Inport  Port=2
  System_On : Inport  Port=3
  In4 : Inport  Port=4
  In5 : Inport  Port=5
  Disable_Audio : Inport  Port=6
  In7 : Inport  Port=7
  In8 : Inport  Port=8
  In9 : Inport  Port=9
  VTBI_High : Inport  Port=10
  In11 : Inport  Port=11
  In12 : Inport  Port=12
  Air_In_Line : Inport  Port=13
  Occlusion : Inport  Port=14
  Door_Open : Inport  Port=15
  In16 : Inport  Port=16
  In17 : Inport  Port=17
  In18 : Inport  Port=18
  In19 : Inport  Port=19
  In20 : Inport  Port=20
  In21 : Inport  Port=21
  In22 : Inport  Port=22
  In23 : Inport  Port=23
  In24 : Inport  Port=24
  In25 : Inport  Port=25
  In26 : Inport  Port=26
  In27 : Inport  Port=27
  In28 : Inport  Port=28
  In29 : Inport  Port=29
  Audio_Level : Inport  Port=30
  In31 : Inport  Port=31
  In32 : Inport  Port=32
  In33 : Inport  Port=33
  In34 : Inport  Port=34
  In35 : Inport  Port=35
  In36 : Inport  Port=36
  In37 : Inport  Port=37
  In38 : Inport  Port=38
  Reservoir_Empty : Inport  Port=39
  In40 : Inport  Port=40
  Volume_Infused : Inport  Port=41
  In_Therapy : Inport  Port=42
  In43 : Inport  Port=43
  Is_Audio_Disabled : Inport  Port=44
  Audio_Notification_Command : Inport  Port=45
  Highest_Level_Alarm : Inport  Port=46
  Air_In_Line_term : Terminator
  Compare To Constant : simulink/Logic and Bit Operations/Compare To Constant  relop===  const=0  OutDataTypeStr=boolean
  Compare To Constant1 : simulink/Logic and Bit Operations/Compare To Constant  relop=>=  const=3.0  OutDataTypeStr=boolean
  Compare To Constant2 : simulink/Logic and Bit Operations/Compare To Constant  relop===  const=0  OutDataTypeStr=boolean
  Door_Open_term : Terminator
  In11_term : Terminator
  In12_term : Terminator
  In16_term : Terminator
  In17_term : Terminator
  In18_term : Terminator
  In19_term : Terminator
  In1_term : Terminator
  In20_term : Terminator
  In21_term : Terminator
  In22_term : Terminator
  In23_term : Terminator
  In24_term : Terminator
  In25_term : Terminator
  In26_term : Terminator
  In27_term : Terminator
  In28_term : Terminator
  In29_term : Terminator
  In2_term : Terminator
  In31_term : Terminator
  In32_term : Terminator
  In33_term : Terminator
  In34_term : Terminator
  In35_term : Terminator
  In36_term : Terminator
  In37_term : Terminator
  In38_term : Terminator
  In40_term : Terminator
  In43_term : Terminator
  In4_term : Terminator
  In5_term : Terminator
  In7_term : Terminator
  In8_term : Terminator
  In9_term : Terminator
  In_Therapy_term : Terminator
  Logical Operator : Logic  Inputs=3  AllPortsSameDT=off  OutDataTypeStr=boolean
  Logical Operator1 : Logic  Operator=NOT  Inputs=3  AllPortsSameDT=off  OutDataTypeStr=boolean
  Logical Operator2 : Logic  Operator=OR  AllPortsSameDT=off  OutDataTypeStr=boolean
  Logical Operator3 : Logic  AllPortsSameDT=off  OutDataTypeStr=boolean
  Memory : Memory
  Occlusion_term : Terminator
  Relational Operator : RelationalOperator  Operator===  OutDataTypeStr=boolean
  Reservoir_Empty_term : Terminator
  VTBI_High_term : Terminator
  Volume_Infused_term : Terminator
  alarm_gte_L3_causes_audio_output_EQ_audio_level : Outport
  wires:
  In1/1 -> In1_term/1
  In2/1 -> In2_term/1
  In4/1 -> In4_term/1
  In5/1 -> In5_term/1
  Disable_Audio/1 -> Compare To Constant2/1
  In7/1 -> In7_term/1
  In8/1 -> In8_term/1
  In9/1 -> In9_term/1
  VTBI_High/1 -> VTBI_High_term/1
  In11/1 -> In11_term/1
  In12/1 -> In12_term/1
  Air_In_Line/1 -> Air_In_Line_term/1
  Occlusion/1 -> Occlusion_term/1
  Door_Open/1 -> Door_Open_term/1
  In16/1 -> In16_term/1
  In17/1 -> In17_term/1
  In18/1 -> In18_term/1
  In19/1 -> In19_term/1
  In20/1 -> In20_term/1
  In21/1 -> In21_term/1
  In22/1 -> In22_term/1
  In23/1 -> In23_term/1
  In24/1 -> In24_term/1
  In25/1 -> In25_term/1
  In26/1 -> In26_term/1
  In27/1 -> In27_term/1
  In28/1 -> In28_term/1
  In29/1 -> In29_term/1
  Audio_Level/1 -> Relational Operator/2
  In31/1 -> In31_term/1
  In32/1 -> In32_term/1
  In33/1 -> In33_term/1
  In34/1 -> In34_term/1
  In35/1 -> In35_term/1
  In36/1 -> In36_term/1
  In37/1 -> In37_term/1
  In38/1 -> In38_term/1
  Reservoir_Empty/1 -> Reservoir_Empty_term/1
  In40/1 -> In40_term/1
  Volume_Infused/1 -> Volume_Infused_term/1
  In_Therapy/1 -> In_Therapy_term/1
  In43/1 -> In43_term/1
  Audio_Notification_Command/1 -> Relational Operator/1
  System_On/1 -> Logical Operator/1
  Highest_Level_Alarm/1 -> Memory/1
  Logical Operator/1 -> Logical Operator1/1
  Logical Operator1/1 -> Logical Operator2/1
  Logical Operator2/1 -> alarm_gte_L3_causes_audio_output_EQ_audio_level/1
  Memory/1 -> Compare To Constant1/1
  Compare To Constant1/1 -> Logical Operator/2
  Compare To Constant2/1 -> Logical Operator/3
  Is_Audio_Disabled/1 -> Compare To Constant/1
  Relational Operator/1 -> Logical Operator3/1
  Compare To Constant/1 -> Logical Operator3/2
  Logical Operator3/1 -> Logical Operator2/2

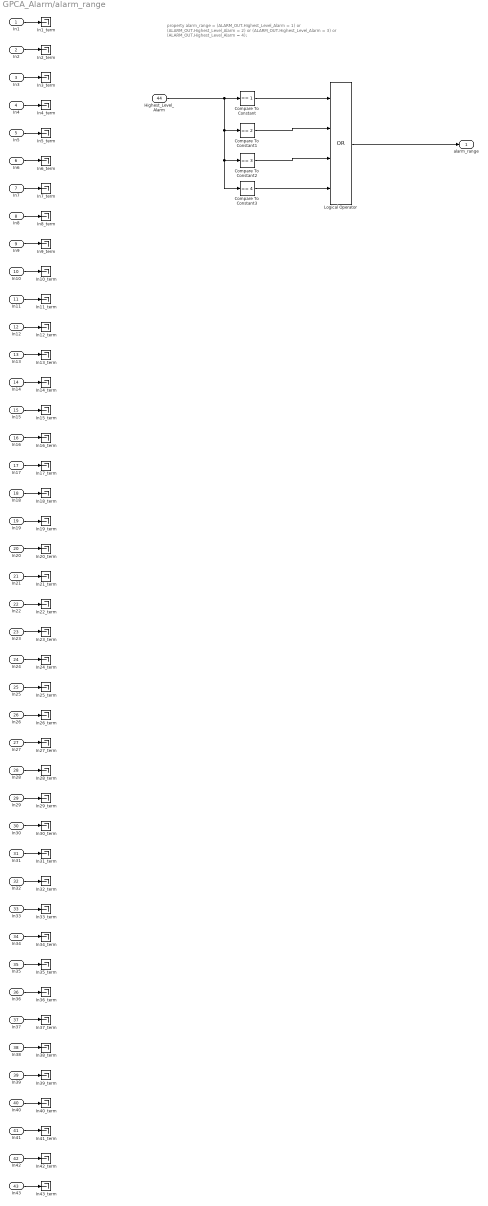
== system GPCA_Alarm/alarm_range ==
  note: property alarm_range =
      | (ALARM_OUT.Highest_Level_Alarm = 1) or
      | (ALARM_OUT.Highest_Level_Alarm = 2) or
      | (ALARM_OUT.Highest_Level_Alarm = 3) or
      | (ALARM_OUT.Highest_Level_Alarm = 4);
  In1 : Inport
  In2 : Inport  Port=2
  In3 : Inport  Port=3
  In4 : Inport  Port=4
  In5 : Inport  Port=5
  In6 : Inport  Port=6
  In7 : Inport  Port=7
  In8 : Inport  Port=8
  In9 : Inport  Port=9
  In10 : Inport  Port=10
  In11 : Inport  Port=11
  In12 : Inport  Port=12
  In13 : Inport  Port=13
  In14 : Inport  Port=14
  In15 : Inport  Port=15
  In16 : Inport  Port=16
  In17 : Inport  Port=17
  In18 : Inport  Port=18
  In19 : Inport  Port=19
  In20 : Inport  Port=20
  In21 : Inport  Port=21
  In22 : Inport  Port=22
  In23 : Inport  Port=23
  In24 : Inport  Port=24
  In25 : Inport  Port=25
  In26 : Inport  Port=26
  In27 : Inport  Port=27
  In28 : Inport  Port=28
  In29 : Inport  Port=29
  In30 : Inport  Port=30
  In31 : Inport  Port=31
  In32 : Inport  Port=32
  In33 : Inport  Port=33
  In34 : Inport  Port=34
  In35 : Inport  Port=35
  In36 : Inport  Port=36
  In37 : Inport  Port=37
  In38 : Inport  Port=38
  In39 : Inport  Port=39
  In40 : Inport  Port=40
  In41 : Inport  Port=41
  In42 : Inport  Port=42
  In43 : Inport  Port=43
  Highest_Level_Alarm : Inport  Port=44
  Compare To Constant : simulink/Logic and Bit Operations/Compare To Constant  relop===  const=1  OutDataTypeStr=boolean
  Compare To Constant1 : simulink/Logic and Bit Operations/Compare To Constant  relop===  const=2  OutDataTypeStr=boolean
  Compare To Constant2 : simulink/Logic and Bit Operations/Compare To Constant  relop===  const=3  OutDataTypeStr=boolean
  Compare To Constant3 : simulink/Logic and Bit Operations/Compare To Constant  relop===  const=4  OutDataTypeStr=boolean
  In10_term : Terminator
  In11_term : Terminator
  In12_term : Terminator
  In13_term : Terminator
  In14_term : Terminator
  In15_term : Terminator
  In16_term : Terminator
  In17_term : Terminator
  In18_term : Terminator
  In19_term : Terminator
  In1_term : Terminator
  In20_term : Terminator
  In21_term : Terminator
  In22_term : Terminator
  In23_term : Terminator
  In24_term : Terminator
  In25_term : Terminator
  In26_term : Terminator
  In27_term : Terminator
  In28_term : Terminator
  In29_term : Terminator
  In2_term : Terminator
  In30_term : Terminator
  In31_term : Terminator
  In32_term : Terminator
  In33_term : Terminator
  In34_term : Terminator
  In35_term : Terminator
  In36_term : Terminator
  In37_term : Terminator
  In38_term : Terminator
  In39_term : Terminator
  In3_term : Terminator
  In40_term : Terminator
  In41_term : Terminator
  In42_term : Terminator
  In43_term : Terminator
  In4_term : Terminator
  In5_term : Terminator
  In6_term : Terminator
  In7_term : Terminator
  In8_term : Terminator
  In9_term : Terminator
  Logical Operator : Logic  Operator=OR  Inputs=4  AllPortsSameDT=off  OutDataTypeStr=boolean
  alarm_range : Outport
  wires:
  In1/1 -> In1_term/1
  In2/1 -> In2_term/1
  In3/1 -> In3_term/1
  In4/1 -> In4_term/1
  In5/1 -> In5_term/1
  In6/1 -> In6_term/1
  In7/1 -> In7_term/1
  In8/1 -> In8_term/1
  In9/1 -> In9_term/1
  In10/1 -> In10_term/1
  In11/1 -> In11_term/1
  In12/1 -> In12_term/1
  In13/1 -> In13_term/1
  In14/1 -> In14_term/1
  In15/1 -> In15_term/1
  In16/1 -> In16_term/1
  In17/1 -> In17_term/1
  In18/1 -> In18_term/1
  In19/1 -> In19_term/1
  In20/1 -> In20_term/1
  In21/1 -> In21_term/1
  In22/1 -> In22_term/1
  In23/1 -> In23_term/1
  In24/1 -> In24_term/1
  In25/1 -> In25_term/1
  In26/1 -> In26_term/1
  In27/1 -> In27_term/1
  In28/1 -> In28_term/1
  In29/1 -> In29_term/1
  In30/1 -> In30_term/1
  In31/1 -> In31_term/1
  In32/1 -> In32_term/1
  In33/1 -> In33_term/1
  In34/1 -> In34_term/1
  In35/1 -> In35_term/1
  In36/1 -> In36_term/1
  In37/1 -> In37_term/1
  In38/1 -> In38_term/1
  In39/1 -> In39_term/1
  In40/1 -> In40_term/1
  In41/1 -> In41_term/1
  In42/1 -> In42_term/1
  In43/1 -> In43_term/1
  Highest_Level_Alarm/1 -> Compare To Constant3/1, Compare To Constant2/1, Compare To Constant1/1, Compare To Constant/1
  Compare To Constant/1 -> Logical Operator/1
  Compare To Constant1/1 -> Logical Operator/2
  Compare To Constant2/1 -> Logical Operator/3
  Compare To Constant3/1 -> Logical Operator/4
  Logical Operator/1 -> alarm_range/1
